simulink model "auv_kinematic1"  (R2018a)
settings: Solver=VariableStepAuto  StartTime=0.0  StopTime=6000  RelTol=1e-3
undefined symbols (not defined in the file or in its folder): Angular, Linear
libraries: robotlib x2, simulink x1
settings Model: Creator=User  LastModifiedBy=allen
settings CodeAppCC: StateflowObjectComments=on

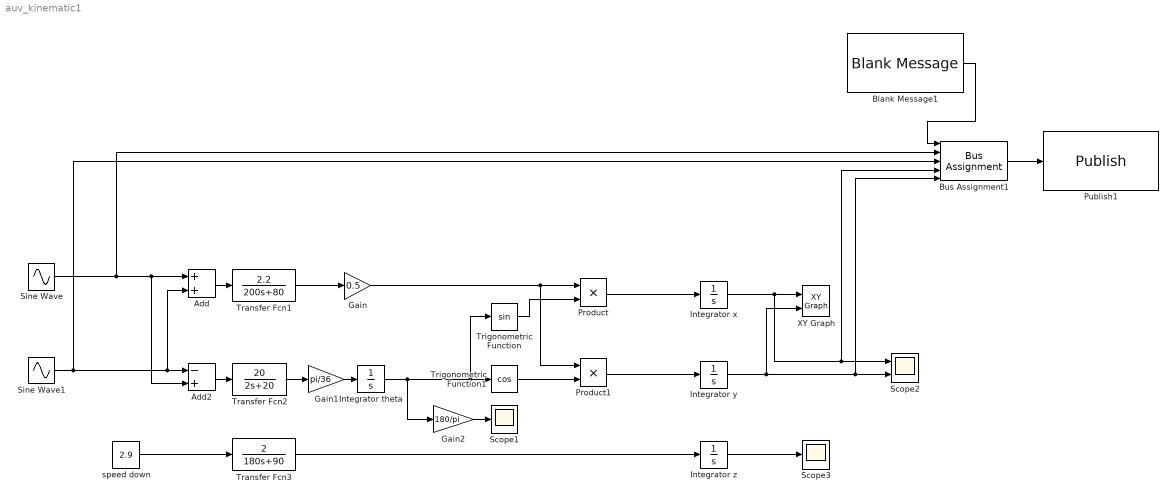
== system auv_kinematic1 ==
  Add : Sum
  Add2 : Sum  Inputs=-+
  Blank Message1 : robotlib/Blank Message  SourceLibraryInfo=This block requires Robotics System Toolbox  messageType=geometry_msgs/Twist  SampleTime=inf
      settings: SourceProductBaseCode=RO
  Bus Assignment1 : BusAssignment  AssignedSignals=Linear.X,Linear.Y,Angular.X,Angular.Y
  Gain : Gain  Gain=0.5
  Gain1 : Gain  Gain=pi/36
  Gain2 : Gain  Gain=180/pi
  Integrator theta : Integrator  InitialCondition=pi/4
  Integrator x : Integrator
  Integrator y : Integrator
  Integrator z : Integrator
  Product : Product
  Product1 : Product
  Publish1 : robotlib/Publish  SourceLibraryInfo=This block requires Robotics System Toolbox  topicSource=Specify your own  topic=/Asv_traindata  messageType=geometry_msgs/Twist  messageQueueLength=1
      settings: SourceProductBaseCode=RO
  Scope1 : Scope
  Scope2 : Scope  NumInputPorts=2
  Scope3 : Scope
  Sine Wave : Sin  Frequency=0.01  Phase=pi  SampleTime=0
  Sine Wave1 : Sin  Frequency=0.05  SampleTime=0
  Transfer Fcn1 : TransferFcn  Numerator=2.2  Denominator=[200 80]
  Transfer Fcn2 : TransferFcn  Numerator=20  Denominator=[2 20]
  Transfer Fcn3 : TransferFcn  Numerator=2  Denominator=[180 90]
  Trigonometric Function : Trigonometry
  Trigonometric Function1 : Trigonometry  Operator=cos
  XY Graph : simulink/Sinks/XY Graph  xmin=-20  xmax=20  ymin=-20  ymax=20  st=-1
  speed down : Constant  Value=2.9
  wires:
  Trigonometric Function/1 -> Product/2
  Trigonometric Function1/1 -> Product1/2
  Product1/1 -> Integrator y/1
  Integrator y/1 -> Bus Assignment1/5, Scope2/2, XY Graph/2
  Gain/1 -> Product1/1, Product/1
  Gain1/1 -> Integrator theta/1
  Integrator theta/1 -> Gain2/1, Trigonometric Function/1, Trigonometric Function1/1
  Product/1 -> Integrator x/1
  Add/1 -> Transfer Fcn1/1
  Transfer Fcn1/1 -> Gain/1
  Add2/1 -> Transfer Fcn2/1
  Transfer Fcn2/1 -> Gain1/1
  speed down/1 -> Transfer Fcn3/1
  Transfer Fcn3/1 -> Integrator z/1
  Integrator z/1 -> Scope3/1
  Gain2/1 -> Scope1/1
  Blank Message1/1 -> Bus Assignment1/1
  Integrator x/1 -> Bus Assignment1/4, Scope2/1, XY Graph/1
  Sine Wave/1 -> Bus Assignment1/2, Add2/2, Add/1
  Bus Assignment1/1 -> Publish1/1
  Sine Wave1/1 -> Add2/1, Add/2, Bus Assignment1/3
